simulink model "AA_Assemblage"  (R2020b)
settings: Solver=FixedStepAuto  StartTime=0.0  StopTime=inf  FixedStep=0.001  RelTol=1e-3
values from neighbouring files (symbols this model uses):
  smiData =     [A_robot_move.mat]
undefined symbols (not defined in the file or in its folder): Levenberg, Marquardt, W, X, Y, Z
libraries: sm_lib x1154, nesl_utility x40, robotlib x9, robotmaniplib x4, robotcorelib x2, simulink x1
(part 1 of 19)
settings Model: Creator=alessandrini  LastModifiedBy=alessandrini

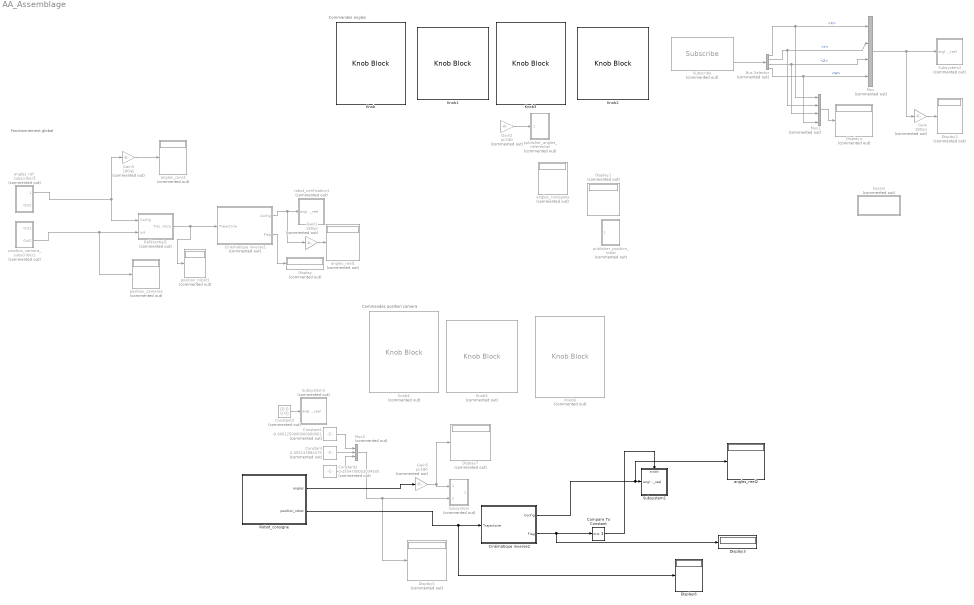
== system AA_Assemblage ==
  note: Fonctionnement global
  note: Commandes angles
  note: Commandes position camera
  Bus Selector : BusSelector  Commented=on  OutputSignals=X,Y,Z,W
  Cinématique inverse1 : Subsystem  Commented=on
  Cinématique inverse2 : Subsystem
  Compare To Constant : simulink/Logic and Bit Operations/Compare To Constant  relop===  const=1  OutDataTypeStr=boolean
  Constant : Constant  Commented=on  Value=0.055133984375
  Constant1 : Constant  Commented=on  Value=-0.0001250000000000001
  Constant2 : Constant  Commented=on  Value=0.1554700002034505
  Constant3 : Constant  Commented=on  Value=[0 0 0 0]
  Display{,1..2,4..5,7} (6 alike) : Display  Commented=on
  Display3 : Display
  Display6 : Display
  Gain : Gain  Commented=on  Gain=180/pi
  Gain1 : Gain  Commented=on  Gain=180/pi
  Gain2 : Gain  Commented=on  Gain=pi/180
  Gain3 : Gain  Commented=on  Gain=180/pi
  Gain5 : Gain  Commented=on  Gain=pi/180
  Knob : KnobBlock  ScaleMin=-30  ScaleMax=115
  Knob1 : KnobBlock  ScaleMin=-90  ScaleMax=45
  Knob2 : KnobBlock  ScaleMin=-60  ScaleMax=0
  Knob3 : KnobBlock  ScaleMin=-90  ScaleMax=20
  Knob4 : KnobBlock  Commented=on  ScaleMin=-0.01  ScaleMax=0.01
  Knob5 : KnobBlock  Commented=on  ScaleMin=0.05  ScaleMax=0.06
  Knob6 : KnobBlock  Commented=on  ScaleMin=0.15  ScaleMax=0.16
  Mux : Mux  Commented=on
  Mux1 : Mux  Commented=on
  Mux2 : Mux  Commented=on  Inputs=3
  Robot_consigne : Subsystem
  Référentiel1 : Subsystem  Commented=on
  Subscribe : robotlib/Subscribe  Commented=on  topicSource=Specify your own  topic=/angles_liaison  messageType=geometry_msgs/Quaternion  SampleTime=-1  legacyBusStruct=off  messageQueueLength=1
  Subsystem : Subsystem  Commented=on
  Subsystem1 : Subsystem
  Subsystem2 : Subsystem  Commented=on
  Subsystem3 : Subsystem  Commented=on
  angles_cons1 : Display  Commented=on
  angles_consignes : Display  Commented=on
  angles_reel1 : Display  Commented=on
  angles_reel2 : Display
  angles_ref_subscriber1 : Subsystem  Commented=on
  bassin : Subsystem  Commented=on  TreatAsAtomicUnit=on
  position_camera1 : Display  Commented=on
  position_camera_subscriber1 : Subsystem  Commented=on
  position_robot1 : Display  Commented=on
  publisher_angles_referentiel : Subsystem  Commented=on
  publisher_position_robot : Subsystem  Commented=on
  robot_verification1 : Subsystem  Commented=on
  wires:
  Gain1/1 -> angles_reel1/1
  Cinématique inverse1/2(Flag) -> Display/1
  Gain2/1 -> publisher_angles_referentiel/1(position)
  Cinématique inverse1/1(Config) -> Gain1/1, robot_verification1/1(angles_reel)
  Référentiel1/1(Trajectoire) -> Cinématique inverse1/1(Trajectoire), position_robot1/1
  position_camera_subscriber1/2(Out2) -> position_camera1/1, Référentiel1/2(In3)
  Gain3/1 -> angles_cons1/1
  angles_ref_subscriber1/1(Config) -> Gain3/1, Référentiel1/1(Config)
  Subscribe/2 -> Bus Selector/1
  Bus Selector/1 -> Mux1/1, Mux/1  "<X>"
  Bus Selector/4 -> Mux1/4, Mux/4  "<W>"
  Mux/1 -> Subsystem2/1(angles_reel), Gain/1
  Bus Selector/2 -> Mux/2, Mux1/2  "<Y>"
  Bus Selector/3 -> Mux/3, Mux1/3  "<Z>"
  Cinématique inverse2/1(Config) -> Subsystem1/1(angles_reel), angles_reel2/1
  Mux1/1 -> Display4/1
  Gain/1 -> Display2/1
  Cinématique inverse2/2(Flag) -> Display3/1, Compare To Constant/1
  Gain5/1 -> Display7/1, Subsystem/1(Config)
  Mux2/1 -> Display5/1, Subsystem/2(position)
  Constant/1 -> Mux2/2
  Constant1/1 -> Mux2/1
  Constant2/1 -> Mux2/3
  Constant3/1 -> Subsystem3/1(angles_reel)
  Robot_consigne/1(angles) -> Gain5/1
  Robot_consigne/2(position_robot) -> Display6/1, Cinématique inverse2/1(Trajectoire)
  Compare To Constant/1 -> Subsystem1/Enable

== system AA_Assemblage/Cinématique inverse1 ==
  Trajectoire : Inport
  Bus Selector : BusSelector  OutputSignals=ExitFlag
  Constant1 : Constant  Value=[0 0 0 1 1 1]  VectorParams1D=off
  Coordinate Transformation Conversion1 : robotcorelib/Coordinate Transformation Conversion  InputRepresentation=Translation Vector  InputEulerSequence=ZYX  ShowTrVecInputPort=on  OutputRepresentation=Homogeneous Transformation  OutputEulerSequence=ZYX  ShowTrVecOutputPort=on  SimulateUsing=Interpreted execution
  Delay : Delay  DelayLength=1  InitialCondition=([-45.92 243 205.5 63.6]*pi/180)'
  Inverse Kinematics : robotmaniplib/Inverse Kinematics  RigidBodyTree=robot  EndEffector=Body5  ShowInfo=on  SolverName=Levenberg-Marquardt  EnforceJointLimits=on  MaxIterations=1500  MaxTime=10  GradientTolerance=1e-7  SolutionTolerance=1e-6  StepTolerance=1e-14  ErrorChangeTolerance=1e-12  UseErrorDamping=on  DampingBias=0.0025  SimulateUsing=Interpreted execution
  Config : Outport
  Flag : Outport  Port=2
  wires:
  Coordinate Transformation Conversion1/1 -> Inverse Kinematics/1
  Delay/1 -> Inverse Kinematics/3
  Constant1/1 -> Inverse Kinematics/2
  Trajectoire/1 -> Coordinate Transformation Conversion1/1
  Inverse Kinematics/1 -> Delay/1, Config/1
  Inverse Kinematics/2 -> Bus Selector/1
  Bus Selector/1 -> Flag/1  "<ExitFlag>"

== system AA_Assemblage/Cinématique inverse2 ==
  Trajectoire : Inport
  Bus Selector : BusSelector  OutputSignals=ExitFlag
  Constant1 : Constant  Value=[0 0 0 1 1 1]  VectorParams1D=off
  Coordinate Transformation Conversion1 : robotcorelib/Coordinate Transformation Conversion  InputRepresentation=Translation Vector  InputEulerSequence=ZYX  ShowTrVecInputPort=on  OutputRepresentation=Homogeneous Transformation  OutputEulerSequence=ZYX  ShowTrVecOutputPort=on  SimulateUsing=Interpreted execution
  Delay1 : Delay  DelayLength=1  InitialCondition=([19 43 0 -30]*pi/180)'
  Inverse Kinematics : robotmaniplib/Inverse Kinematics  RigidBodyTree=robot  EndEffector=Body5  ShowInfo=on  SolverName=Levenberg-Marquardt  EnforceJointLimits=on  MaxIterations=1500  MaxTime=10  GradientTolerance=1e-7  SolutionTolerance=1e-6  StepTolerance=1e-14  ErrorChangeTolerance=1e-12  UseErrorDamping=on  DampingBias=0.0025  SimulateUsing=Interpreted execution
  Config : Outport
  Flag : Outport  Port=2
  wires:
  Coordinate Transformation Conversion1/1 -> Inverse Kinematics/1
  Delay1/1 -> Inverse Kinematics/3
  Constant1/1 -> Inverse Kinematics/2
  Trajectoire/1 -> Coordinate Transformation Conversion1/1
  Inverse Kinematics/1 -> Delay1/1, Config/1
  Inverse Kinematics/2 -> Bus Selector/1
  Bus Selector/1 -> Flag/1  "<ExitFlag>"

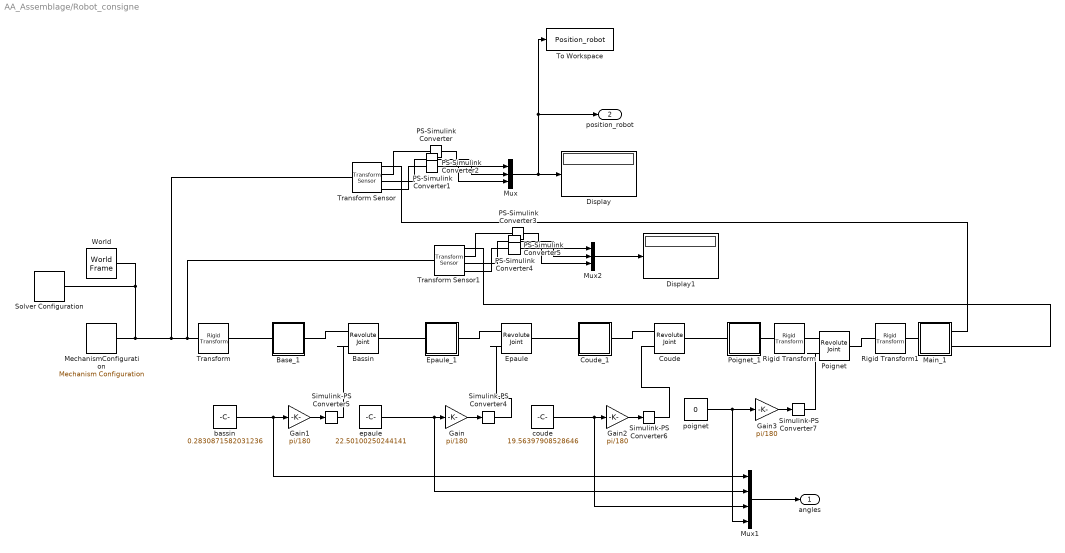
== system AA_Assemblage/Robot_consigne ==
  Base_1 : Subsystem
  Bassin : sm_lib/Joints/Revolute Joint  JointMode=Normal  SenseConstraintForce=off  SenseConstraintForceX=off  SenseConstraintForceY=off  SenseConstraintForceZ=off  SenseConstraintTorque=off  SenseConstraintTorqueX=off  SenseConstraintTorqueY=off  SenseConstraintTorqueZ=off  SenseTotalForce=off  SenseTotalForceX=off  SenseTotalForceY=off  SenseTotalForceZ=off  SenseTotalTorque=off  SenseTotalTorqueX=off  SenseTotalTorqueY=off  SenseTotalTorqueZ=off  CompositeWrenchDir=FollowerOnBase  CompositeWrenchFrame=BaseFrame  EquilibriumPosition=0  EquilibriumPositionUnits=deg  SpringStiffness=0  SpringStiffnessUnits=N*m/deg  DampingCoefficient=0  DampingCoefficientUnits=N*m/(deg/s)  TorqueActuationMode=ComputedTorque  MotionActuationMode=InputMotion  SensePosition=off  SenseVelocity=off  SenseAcceleration=off  SenseTorqueForce=off  SenseLowerLimitTorqueForce=off  SenseUpperLimitTorqueForce=off  LowerLimitSpecify=off  LowerLimitBound=-90  LowerLimitBoundUnits=deg  LowerLimitStiffness=1e4  LowerLimitStiffnessUnits=N*m/deg  LowerLimitDamping=10  LowerLimitDampingUnits=N*m/(deg/s)  LowerLimitTransitionRegionWidth=0.1  LowerLimitTransitionRegionWidthUnits=deg  UpperLimitSpecify=off  UpperLimitBound=90  UpperLimitBoundUnits=deg  UpperLimitStiffness=1e4  UpperLimitStiffnessUnits=N*m/deg  UpperLimitDamping=10  UpperLimitDampingUnits=N*m/(deg/s)  UpperLimitTransitionRegionWidth=0.1  UpperLimitTransitionRegionWidthUnits=deg  PositionTargetSpecify=on  PositionTargetPriority=Low  PositionTargetValue=smiData.RevoluteJoint(4).Rz.Pos  PositionTargetValueUnits=deg  VelocityTargetSpecify=off  VelocityTargetPriority=High  VelocityTargetValue=0  VelocityTargetValueUnits=deg/s
  Coude : sm_lib/Joints/Revolute Joint  JointMode=Normal  SenseConstraintForce=off  SenseConstraintForceX=off  SenseConstraintForceY=off  SenseConstraintForceZ=off  SenseConstraintTorque=off  SenseConstraintTorqueX=off  SenseConstraintTorqueY=off  SenseConstraintTorqueZ=off  SenseTotalForce=off  SenseTotalForceX=off  SenseTotalForceY=off  SenseTotalForceZ=off  SenseTotalTorque=off  SenseTotalTorqueX=off  SenseTotalTorqueY=off  SenseTotalTorqueZ=off  CompositeWrenchDir=FollowerOnBase  CompositeWrenchFrame=BaseFrame  EquilibriumPosition=0  EquilibriumPositionUnits=deg  SpringStiffness=0  SpringStiffnessUnits=N*m/deg  DampingCoefficient=0  DampingCoefficientUnits=N*m/(deg/s)  TorqueActuationMode=ComputedTorque  MotionActuationMode=InputMotion  SensePosition=off  SenseVelocity=off  SenseAcceleration=off  SenseTorqueForce=off  SenseLowerLimitTorqueForce=off  SenseUpperLimitTorqueForce=off  LowerLimitSpecify=off  LowerLimitBound=-90  LowerLimitBoundUnits=deg  LowerLimitStiffness=1e4  LowerLimitStiffnessUnits=N*m/deg  LowerLimitDamping=10  LowerLimitDampingUnits=N*m/(deg/s)  LowerLimitTransitionRegionWidth=0.1  LowerLimitTransitionRegionWidthUnits=deg  UpperLimitSpecify=off  UpperLimitBound=90  UpperLimitBoundUnits=deg  UpperLimitStiffness=1e4  UpperLimitStiffnessUnits=N*m/deg  UpperLimitDamping=10  UpperLimitDampingUnits=N*m/(deg/s)  UpperLimitTransitionRegionWidth=0.1  UpperLimitTransitionRegionWidthUnits=deg  PositionTargetSpecify=on  PositionTargetPriority=Low  PositionTargetValue=smiData.RevoluteJoint(1).Rz.Pos  PositionTargetValueUnits=deg  VelocityTargetSpecify=off  VelocityTargetPriority=High  VelocityTargetValue=0  VelocityTargetValueUnits=deg/s
  Coude_1 : Subsystem
  Display : Display
  Display1 : Display
  Epaule : sm_lib/Joints/Revolute Joint  JointMode=Normal  SenseConstraintForce=off  SenseConstraintForceX=off  SenseConstraintForceY=off  SenseConstraintForceZ=off  SenseConstraintTorque=off  SenseConstraintTorqueX=off  SenseConstraintTorqueY=off  SenseConstraintTorqueZ=off  SenseTotalForce=off  SenseTotalForceX=off  SenseTotalForceY=off  SenseTotalForceZ=off  SenseTotalTorque=off  SenseTotalTorqueX=off  SenseTotalTorqueY=off  SenseTotalTorqueZ=off  CompositeWrenchDir=FollowerOnBase  CompositeWrenchFrame=BaseFrame  EquilibriumPosition=0  EquilibriumPositionUnits=deg  SpringStiffness=0  SpringStiffnessUnits=N*m/deg  DampingCoefficient=0  DampingCoefficientUnits=N*m/(deg/s)  TorqueActuationMode=ComputedTorque  MotionActuationMode=InputMotion  SensePosition=off  SenseVelocity=off  SenseAcceleration=off  SenseTorqueForce=off  SenseLowerLimitTorqueForce=off  SenseUpperLimitTorqueForce=off  LowerLimitSpecify=off  LowerLimitBound=-90  LowerLimitBoundUnits=deg  LowerLimitStiffness=1e4  LowerLimitStiffnessUnits=N*m/deg  LowerLimitDamping=10  LowerLimitDampingUnits=N*m/(deg/s)  LowerLimitTransitionRegionWidth=0.1  LowerLimitTransitionRegionWidthUnits=deg  UpperLimitSpecify=off  UpperLimitBound=90  UpperLimitBoundUnits=deg  UpperLimitStiffness=1e4  UpperLimitStiffnessUnits=N*m/deg  UpperLimitDamping=10  UpperLimitDampingUnits=N*m/(deg/s)  UpperLimitTransitionRegionWidth=0.1  UpperLimitTransitionRegionWidthUnits=deg  PositionTargetSpecify=on  PositionTargetPriority=Low  PositionTargetValue=smiData.RevoluteJoint(3).Rz.Pos  PositionTargetValueUnits=deg  VelocityTargetSpecify=off  VelocityTargetPriority=High  VelocityTargetValue=0  VelocityTargetValueUnits=deg/s
  Epaule_1 : Subsystem
  Gain{,1..3} (4 alike) : Gain  Gain=pi/180
  Main_1 : Subsystem
  MechanismConfiguration : sm_lib/Utilities/Mechanism Configuration  UniformGravity=Constant  GravityVector=[0 0 -9.80665]  GravityVectorUnits=m/s^2  GravityUnits=m/s^2  LinearizationDelta=0.001  JointModeTransitionNonlinearIterations=2
  Mux : Mux  Inputs=3
  Mux1 : Mux
  Mux2 : Mux  Inputs=3
  PS-Simulink Converter{,1..5} (6 alike) : nesl_utility/PS-Simulink Converter  PhysicalDomain=network_engine_domain  SubClassName=ps_output  LeftPortType=input  RightPortType=output  PseudoPeriodic=off  Frequencies=[]  Unit=inherit  AffineConversion=off
  Poignet : sm_lib/Joints/Revolute Joint  JointMode=Normal  SenseConstraintForce=off  SenseConstraintForceX=off  SenseConstraintForceY=off  SenseConstraintForceZ=off  SenseConstraintTorque=off  SenseConstraintTorqueX=off  SenseConstraintTorqueY=off  SenseConstraintTorqueZ=off  SenseTotalForce=off  SenseTotalForceX=off  SenseTotalForceY=off  SenseTotalForceZ=off  SenseTotalTorque=off  SenseTotalTorqueX=off  SenseTotalTorqueY=off  SenseTotalTorqueZ=off  CompositeWrenchDir=FollowerOnBase  CompositeWrenchFrame=BaseFrame  EquilibriumPosition=0  EquilibriumPositionUnits=deg  SpringStiffness=0  SpringStiffnessUnits=N*m/deg  DampingCoefficient=0  DampingCoefficientUnits=N*m/(deg/s)  TorqueActuationMode=ComputedTorque  MotionActuationMode=InputMotion  SensePosition=off  SenseVelocity=off  SenseAcceleration=off  SenseTorqueForce=off  SenseLowerLimitTorqueForce=off  SenseUpperLimitTorqueForce=off  LowerLimitSpecify=off  LowerLimitBound=-90  LowerLimitBoundUnits=deg  LowerLimitStiffness=1e4  LowerLimitStiffnessUnits=N*m/deg  LowerLimitDamping=10  LowerLimitDampingUnits=N*m/(deg/s)  LowerLimitTransitionRegionWidth=0.1  LowerLimitTransitionRegionWidthUnits=deg  UpperLimitSpecify=off  UpperLimitBound=90  UpperLimitBoundUnits=deg  UpperLimitStiffness=1e4  UpperLimitStiffnessUnits=N*m/deg  UpperLimitDamping=10  UpperLimitDampingUnits=N*m/(deg/s)  UpperLimitTransitionRegionWidth=0.1  UpperLimitTransitionRegionWidthUnits=deg  PositionTargetSpecify=on  PositionTargetPriority=Low  PositionTargetValue=smiData.RevoluteJoint(2).Rz.Pos  PositionTargetValueUnits=deg  VelocityTargetSpecify=off  VelocityTargetPriority=High  VelocityTargetValue=0  VelocityTargetValueUnits=deg/s
  Poignet_1 : Subsystem
  Rigid Transform : sm_lib/Frames and Transforms/Rigid Transform  TranslationMethod=None  TranslationStandardOffset=0  TranslationLengthUnit=m  TranslationStandardAxis=+Z  TranslationCartesianOffset=[0 0 0]  TranslationROffset=0  TranslationROffsetUnits=m  TranslationZOffset=0  TranslationZOffsetUnits=m  TranslationThetaOffset=0  TranslationThetaOffsetUnits=deg  RotationMethod=ArbitraryAxis  RotationAngleUnits=deg  RotationStandardAxis=+Z  RotationAngle=180  RotationArbitraryAxis=[1 0 0]  FollAlignAxisA=+X  BaseAlignAxisA=+Y  FollAlignAxisB=+Y  BaseAlignAxisB=+Z  RotationSequenceAxes=FollowerAxes  RotationSequence=XYX  RotationSequenceAngles=[0 0 0]  RotationSequenceAnglesUnits=deg  RotationMatrix=[1 0 0; 0 1 0; 0 0 1]
  Rigid Transform1 : sm_lib/Frames and Transforms/Rigid Transform  TranslationMethod=None  TranslationStandardOffset=0  TranslationLengthUnit=m  TranslationStandardAxis=+Z  TranslationCartesianOffset=[0 0 0]  TranslationROffset=0  TranslationROffsetUnits=m  TranslationZOffset=0  TranslationZOffsetUnits=m  TranslationThetaOffset=0  TranslationThetaOffsetUnits=deg  RotationMethod=ArbitraryAxis  RotationAngleUnits=deg  RotationStandardAxis=+Z  RotationAngle=180  RotationArbitraryAxis=[1 0 0]  FollAlignAxisA=+X  BaseAlignAxisA=+Y  FollAlignAxisB=+Y  BaseAlignAxisB=+Z  RotationSequenceAxes=FollowerAxes  RotationSequence=XYX  RotationSequenceAngles=[0 0 0]  RotationSequenceAnglesUnits=deg  RotationMatrix=[1 0 0; 0 1 0; 0 0 1]
  Simulink-PS Converter{4..7} (4 alike) : nesl_utility/Simulink-PS Converter  PhysicalDomain=network_engine_domain  SubClassName=ps_input  LeftPortType=input  RightPortType=output  PseudoPeriodic=off  Frequencies=[]  NoiseDistribution=none  NoiseParameters=[]  Unit=1  AffineConversion=off  FilteringAndDerivatives=provide  SimscapeFilterOrder=1  InputFilterTimeConstant=0.001  UdotUserProvided=0
  Solver Configuration : nesl_utility/Solver Configuration  PhysicalDomain=network_engine_domain  SubClassName=solver  LeftPortType=input  RightPortType=generic  Tones=[]  Harmonics=[]  SimulateNoise=off  Profile=off  UseLocalSampling=off  EnableSwitchedLinearOptims=on  FrequencyDomain=off  UseCCode=off  RelTol=0.001  AbsTol=1e-06  MinStep=1e-09  ToWorkspace=off  RevertToSquareIcSolve=off  NumHomotopyIterations=100  PhasorMode=off  PhasorModeNumHarmonics=1  DoDC=off  ResidualTolerance=1e-09  UseLocalSolver=off  LocalSolverChoice=NE_BACKWARD_EULER_ADVANCER  LocalSolverSampleTime=0.001  DoFixedCost=off  MaxNonlinIter=3  MaxModeIter=2  ComputeImpulses=off  ImpulseIterations=2  LinearAlgebra=auto  EquationFormulation=NE_TIME_EF  DelaysMemoryBudget=1024  AutomaticFiltering=on  FilteringTimeConstant=0.001  PartitionStorageMethod=AS_NEEDED  PartitionMemoryBudget=1024  PartitionMethod=ROBUST
  To Workspace : ToWorkspace  VariableName=Position_robot  SaveFormat=Timeseries  SampleTime=-1
  Transform : sm_lib/Frames and Transforms/Rigid Transform  TranslationMethod=Cartesian  TranslationStandardOffset=0  TranslationLengthUnit=mm  TranslationStandardAxis=+Z  TranslationCartesianOffset=smiData.RigidTransform(104).translation  TranslationROffset=0  TranslationROffsetUnits=m  TranslationZOffset=0  TranslationZOffsetUnits=m  TranslationThetaOffset=0  TranslationThetaOffsetUnits=deg  RotationMethod=ArbitraryAxis  RotationAngleUnits=rad  RotationStandardAxis=+Z  RotationAngle=smiData.RigidTransform(104).angle  RotationArbitraryAxis=smiData.RigidTransform(104).axis  FollAlignAxisA=+X  BaseAlignAxisA=+Y  FollAlignAxisB=+Y  BaseAlignAxisB=+Z  RotationSequenceAxes=FollowerAxes  RotationSequence=XYX  RotationSequenceAngles=[0 0 0]  RotationSequenceAnglesUnits=deg  RotationMatrix=[1 0 0; 0 1 0; 0 0 1]
  Transform Sensor : sm_lib/Frames and Transforms/Transform Sensor  MeasurementFrame=World  SenseAngle=off  SenseAxis=off  SenseAngle1=off  SenseAngle2=off  SenseAngle3=off  SenseQ=off  SenseR=off  SenseOmegaX=off  SenseOmegaY=off  SenseOmegaZ=off  SenseOmega1=off  SenseOmega2=off  SenseOmega3=off  SenseQDot=off  SenseRDot=off  SenseAlphaX=off  SenseAlphaY=off  SenseAlphaZ=off  SenseAlpha1=off  SenseAlpha2=off  SenseAlpha3=off  SenseQDDot=off  SenseRDDot=off  SenseX=on  SenseY=on  SenseZ=on  SenseRad=off  SenseAzim=off  SenseDist=off  SenseInc=off  SenseXDot=off  SenseYDot=off  SenseZDot=off  SenseRadDot=off  SenseAzimDot=off  SenseDistDot=off  SenseIncDot=off  SenseXDDot=off  SenseYDDot=off  SenseZDDot=off  SenseRadDDot=off  SenseAzimDDot=off  SenseDistDDot=off  SenseIncDDot=off
  Transform Sensor1 : sm_lib/Frames and Transforms/Transform Sensor  MeasurementFrame=World  SenseAngle=off  SenseAxis=off  SenseAngle1=off  SenseAngle2=off  SenseAngle3=off  SenseQ=off  SenseR=off  SenseOmegaX=off  SenseOmegaY=off  SenseOmegaZ=off  SenseOmega1=off  SenseOmega2=off  SenseOmega3=off  SenseQDot=off  SenseRDot=off  SenseAlphaX=off  SenseAlphaY=off  SenseAlphaZ=off  SenseAlpha1=off  SenseAlpha2=off  SenseAlpha3=off  SenseQDDot=off  SenseRDDot=off  SenseX=on  SenseY=on  SenseZ=on  SenseRad=off  SenseAzim=off  SenseDist=off  SenseInc=off  SenseXDot=off  SenseYDot=off  SenseZDot=off  SenseRadDot=off  SenseAzimDot=off  SenseDistDot=off  SenseIncDot=off  SenseXDDot=off  SenseYDDot=off  SenseZDDot=off  SenseRadDDot=off  SenseAzimDDot=off  SenseDistDDot=off  SenseIncDDot=off
  World : sm_lib/Frames and Transforms/World Frame
  bassin : Constant  Value=0.2830871582031236
  coude : Constant  Value=19.56397908528646
  epaule : Constant  Value=22.50100250244141
  poignet : Constant  Value=0
  angles : Outport
  position_robot : Outport  Port=2
  wires:
  poignet/1 -> Gain3/1, Mux1/4
  bassin/1 -> Mux1/1, Gain1/1
  coude/1 -> Mux1/3, Gain2/1
  Gain/1 -> Simulink-PS Converter4/1
  Gain3/1 -> Simulink-PS Converter7/1
  Gain2/1 -> Simulink-PS Converter6/1
  Gain1/1 -> Simulink-PS Converter5/1
  Mux1/1 -> angles/1
  epaule/1 -> Mux1/2, Gain/1
  PS-Simulink Converter1/1 -> Mux/2
  PS-Simulink Converter/1 -> Mux/1
  PS-Simulink Converter2/1 -> Mux/3
  Mux/1 -> To Workspace/1, position_robot/1, Display/1
  PS-Simulink Converter3/1 -> Mux2/1
  PS-Simulink Converter5/1 -> Mux2/3
  PS-Simulink Converter4/1 -> Mux2/2
  Mux2/1 -> Display1/1
  connections:
  Transform Sensor/LConn1 -- MechanismConfiguration/RConn1 -- Solver Configuration/RConn1 -- World/RConn1 -- Transform Sensor1/LConn1 -- Transform/LConn1
  Transform/RConn1 -- Base_1/LConn1
  Coude/LConn2 -- Simulink-PS Converter6/RConn1
  Base_1/RConn1 -- Bassin/LConn1
  PS-Simulink Converter2/LConn1 -- Transform Sensor/RConn4
  Bassin/LConn2 -- Simulink-PS Converter5/RConn1
  Transform Sensor/RConn1 -- Main_1/RConn1
  PS-Simulink Converter/LConn1 -- Transform Sensor/RConn2
  Poignet/LConn2 -- Simulink-PS Converter7/RConn1
  Poignet/LConn1 -- Rigid Transform/RConn1
  Rigid Transform1/LConn1 -- Poignet/RConn1
  Coude_1/LConn1 -- Epaule/RConn1
  Epaule/LConn1 -- Epaule_1/RConn1
  PS-Simulink Converter1/LConn1 -- Transform Sensor/RConn3
  Coude/LConn1 -- Coude_1/RConn1
  Epaule/LConn2 -- Simulink-PS Converter4/RConn1
  Bassin/RConn1 -- Epaule_1/LConn1
  Coude/RConn1 -- Poignet_1/LConn1
  Main_1/LConn1 -- Rigid Transform1/RConn1
  Rigid Transform/LConn1 -- Poignet_1/RConn1
  PS-Simulink Converter4/LConn1 -- Transform Sensor1/RConn3
  PS-Simulink Converter5/LConn1 -- Transform Sensor1/RConn4
  Main_1/RConn2 -- Transform Sensor1/RConn1
  PS-Simulink Converter3/LConn1 -- Transform Sensor1/RConn2

== system AA_Assemblage/Référentiel1 ==
  Config : Inport
  In3 : Inport  Port=2
  Constant4 : Constant
  Get Transform : robotmaniplib/Get Transform  RigidBodyTree=robot  SourceBody=Body5  TargetBody=Base  SimulateUsing=Interpreted execution
  Mux2 : Mux  Inputs=2
  Product : Product  Multiplication=Matrix(*)
  Selector : Selector  InputPortWidth=4  IndexOptions=Starting index (dialog)  Indices=1  OutputSizes=3
  Trajectoire : Outport
  wires:
  Config/1 -> Get Transform/1
  Constant4/1 -> Mux2/2
  Product/1 -> Selector/1
  In3/1 -> Mux2/1
  Selector/1 -> Trajectoire/1
  Get Transform/1 -> Product/1
  Mux2/1 -> Product/2

== system AA_Assemblage/Subsystem ==
  Config : Inport
  position : Inport  Port=2
  Constant : Constant
  Get Transform : robotmaniplib/Get Transform  RigidBodyTree=robot  SourceBody=Body6  TargetBody=Base  SimulateUsing=Interpreted execution
  Mux : Mux  Inputs=2
  Product : Product  Multiplication=Matrix(*)
  Selector : Selector  InputPortWidth=4  IndexOptions=Starting index (dialog)  Indices=[1]  OutputSizes=3
  Trajectoire : Outport
  wires:
  Selector/1 -> Trajectoire/1
  Product/1 -> Selector/1
  Config/1 -> Get Transform/1
  Get Transform/1 -> Product/1
  position/1 -> Mux/1
  Constant/1 -> Mux/2
  Mux/1 -> Product/2

== system AA_Assemblage/Subsystem1 ==
  note: robot_verification
  angles_reel : Inport
  Enable : EnablePort
  Demux : Demux
  Robot_verif : Subsystem
  Simulink-PS Converter{,1..3} (4 alike) : nesl_utility/Simulink-PS Converter  PhysicalDomain=network_engine_domain  SubClassName=ps_input  LeftPortType=input  RightPortType=output  PseudoPeriodic=off  Frequencies=[]  NoiseDistribution=none  NoiseParameters=[]  Unit=1  AffineConversion=off  FilteringAndDerivatives=filter  SimscapeFilterOrder=2  InputFilterTimeConstant=0.001  UdotUserProvided=0
  wires:
  Demux/2 -> Simulink-PS Converter1/1  "epaule"
  angles_reel/1 -> Demux/1
  Demux/4 -> Simulink-PS Converter3/1  "poignet"
  Demux/1 -> Simulink-PS Converter/1  "bassin"
  Demux/3 -> Simulink-PS Converter2/1  "coude"
  connections:
  Simulink-PS Converter2/RConn1 -- Robot_verif/LConn3
  Simulink-PS Converter1/RConn1 -- Robot_verif/LConn2
  Simulink-PS Converter3/RConn1 -- Robot_verif/LConn4
  Simulink-PS Converter/RConn1 -- Robot_verif/LConn1

== system AA_Assemblage/Subsystem2 ==
  note: robot_verification
  angles_reel : Inport
  Demux : Demux
  Robot_verif : Subsystem
  Simulink-PS Converter{,1..3} (4 alike) : nesl_utility/Simulink-PS Converter  PhysicalDomain=network_engine_domain  SubClassName=ps_input  LeftPortType=input  RightPortType=output  PseudoPeriodic=off  Frequencies=[]  NoiseDistribution=none  NoiseParameters=[]  Unit=1  AffineConversion=off  FilteringAndDerivatives=filter  SimscapeFilterOrder=2  InputFilterTimeConstant=0.001  UdotUserProvided=0
  wires:
  Demux/2 -> Simulink-PS Converter1/1  "epaule"
  angles_reel/1 -> Demux/1
  Demux/4 -> Simulink-PS Converter3/1  "poignet"
  Demux/1 -> Simulink-PS Converter/1  "bassin"
  Demux/3 -> Simulink-PS Converter2/1  "coude"
  connections:
  Simulink-PS Converter2/RConn1 -- Robot_verif/LConn3
  Simulink-PS Converter1/RConn1 -- Robot_verif/LConn2
  Simulink-PS Converter3/RConn1 -- Robot_verif/LConn4
  Simulink-PS Converter/RConn1 -- Robot_verif/LConn1

== system AA_Assemblage/Subsystem3 ==
  note: robot_verification
  angles_reel : Inport
  Demux : Demux
  Robot_verif : Subsystem
  Simulink-PS Converter{,1..3} (4 alike) : nesl_utility/Simulink-PS Converter  PhysicalDomain=network_engine_domain  SubClassName=ps_input  LeftPortType=input  RightPortType=output  PseudoPeriodic=off  Frequencies=[]  NoiseDistribution=none  NoiseParameters=[]  Unit=1  AffineConversion=off  FilteringAndDerivatives=filter  SimscapeFilterOrder=2  InputFilterTimeConstant=0.001  UdotUserProvided=0
  wires:
  Demux/2 -> Simulink-PS Converter1/1  "epaule"
  angles_reel/1 -> Demux/1
  Demux/4 -> Simulink-PS Converter3/1  "poignet"
  Demux/1 -> Simulink-PS Converter/1  "bassin"
  Demux/3 -> Simulink-PS Converter2/1  "coude"
  connections:
  Simulink-PS Converter2/RConn1 -- Robot_verif/LConn3
  Simulink-PS Converter1/RConn1 -- Robot_verif/LConn2
  Simulink-PS Converter3/RConn1 -- Robot_verif/LConn4
  Simulink-PS Converter/RConn1 -- Robot_verif/LConn1

== system AA_Assemblage/angles_ref_subscriber1 ==
  Bus Selector : BusSelector  OutputSignals=X,Y,Z,W
  Mux1 : Mux
  Subscribe : robotlib/Subscribe  topicSource=Specify your own  topic=/angles_ref  messageType=geometry_msgs/Quaternion  SampleTime=-1  legacyBusStruct=off  messageQueueLength=1
  Config : Outport
  Out2 : Outport  Port=2
  wires:
  Subscribe/2 -> Bus Selector/1
  Bus Selector/1 -> Mux1/1  "<X>"
  Bus Selector/2 -> Mux1/2  "<Y>"
  Mux1/1 -> Config/1
  Bus Selector/3 -> Mux1/3  "<Z>"
  Subscribe/1 -> Out2/1
  Bus Selector/4 -> Mux1/4  "<W>"

== system AA_Assemblage/bassin ==
  Add : Sum
  Constant : Constant  Value=-30
  For Iterator : ForIterator  ResetStates=reset  IterationLimit=7
  Gain : Gain  Gain=20
  epaule : Subsystem  TreatAsAtomicUnit=on
  wires:
  Constant/1 -> Add/2
  Add/1 -> epaule/1(In1)
  Gain/1 -> Add/1
  For Iterator/1 -> Gain/1

== system AA_Assemblage/position_camera_subscriber1 ==
  Bus Selector1 : BusSelector  OutputSignals=X,Y,Z
  Mux2 : Mux  Inputs=3
  Subscribe1 : robotlib/Subscribe  topicSource=Specify your own  topic=/position_camera  messageType=geometry_msgs/Point  SampleTime=-1  legacyBusStruct=off  messageQueueLength=1
  Out1 : Outport
  Out2 : Outport  Port=2
  wires:
  Bus Selector1/2 -> Mux2/2  "<Y>"
  Bus Selector1/1 -> Mux2/1  "<X>"
  Subscribe1/2 -> Bus Selector1/1
  Subscribe1/1 -> Out1/1
  Mux2/1 -> Out2/1
  Bus Selector1/3 -> Mux2/3  "<Z>"

== system AA_Assemblage/publisher_angles_referentiel ==
  position : Inport
  Blank Message1 : robotlib/Blank Message  messageClass=Message  entityType=geometry_msgs/Quaternion  messageType=geometry_msgs/Quaternion  SampleTime=inf  legacyBusStruct=off
  Bus Assignment : BusAssignment  AssignedSignals=X,Y,Z,W
  Demux : Demux
  Publish : robotlib/Publish  topicSource=Specify your own  topic=/angles_referentiel  messageType=geometry_msgs/Quaternion  legacyBusStruct=off  messageQueueLength=1
  wires:
  Demux/2 -> Bus Assignment/3
  Bus Assignment/1 -> Publish/1
  Demux/1 -> Bus Assignment/2
  Blank Message1/1 -> Bus Assignment/1
  position/1 -> Demux/1
  Demux/3 -> Bus Assignment/4
  Demux/4 -> Bus Assignment/5

== system AA_Assemblage/publisher_position_robot ==
  position : Inport
  Blank Message1 : robotlib/Blank Message  messageClass=Message  entityType=geometry_msgs/Point  messageType=geometry_msgs/Point  SampleTime=inf  legacyBusStruct=off
  Bus Assignment : BusAssignment  AssignedSignals=X,Y,Z
  Demux : Demux  Outputs=3
  Publish : robotlib/Publish  topicSource=Specify your own  topic=/position_robot  messageType=geometry_msgs/Point  legacyBusStruct=off  messageQueueLength=1
  wires:
  Demux/2 -> Bus Assignment/3
  Bus Assignment/1 -> Publish/1
  Demux/1 -> Bus Assignment/2
  Blank Message1/1 -> Bus Assignment/1
  position/1 -> Demux/1
  Demux/3 -> Bus Assignment/4

== system AA_Assemblage/robot_verification1 ==
  note: robot verification
  angles_reel : Inport
  Demux : Demux
  Robot_verif : Subsystem
  Simulink-PS Converter{,1..3} (4 alike) : nesl_utility/Simulink-PS Converter  PhysicalDomain=network_engine_domain  SubClassName=ps_input  LeftPortType=input  RightPortType=output  PseudoPeriodic=off  Frequencies=[]  NoiseDistribution=none  NoiseParameters=[]  Unit=1  AffineConversion=off  FilteringAndDerivatives=filter  SimscapeFilterOrder=2  InputFilterTimeConstant=0.001  UdotUserProvided=0
  wires:
  Demux/3 -> Simulink-PS Converter2/1  "coude"
  Demux/1 -> Simulink-PS Converter/1  "bassin"
  Demux/4 -> Simulink-PS Converter3/1  "poignet"
  angles_reel/1 -> Demux/1
  Demux/2 -> Simulink-PS Converter1/1  "epaule"
  connections:
  Simulink-PS Converter/RConn1 -- Robot_verif/LConn1
  Simulink-PS Converter3/RConn1 -- Robot_verif/LConn4
  Simulink-PS Converter1/RConn1 -- Robot_verif/LConn2
  Simulink-PS Converter2/RConn1 -- Robot_verif/LConn3

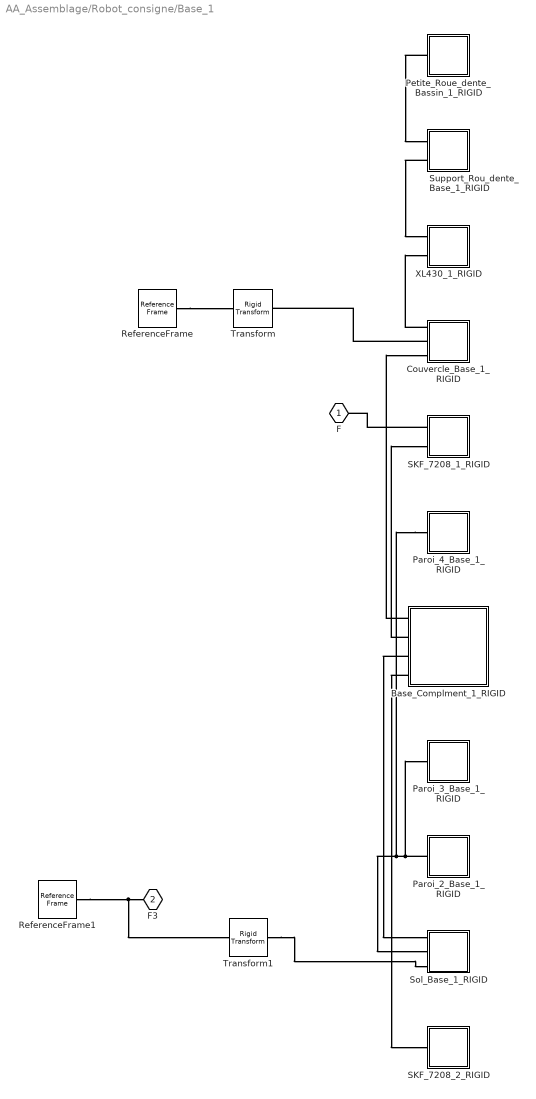
== system AA_Assemblage/Robot_consigne/Base_1 ==
  Base_Complment_1_RIGID : Subsystem
  Couvercle_Base_1_RIGID : Subsystem
  Paroi_2_Base_1_RIGID : Subsystem
  Paroi_3_Base_1_RIGID : Subsystem
  Paroi_4_Base_1_RIGID : Subsystem
  Petite_Roue_dente_Bassin_1_RIGID : Subsystem
  ReferenceFrame : sm_lib/Frames and Transforms/Reference Frame
  ReferenceFrame1 : sm_lib/Frames and Transforms/Reference Frame
  SKF_7208_1_RIGID : Subsystem
  SKF_7208_2_RIGID : Subsystem
  Sol_Base_1_RIGID : Subsystem
  Support_Rou_dente_Base_1_RIGID : Subsystem
  Transform : sm_lib/Frames and Transforms/Rigid Transform  TranslationMethod=Cartesian  TranslationStandardOffset=0  TranslationLengthUnit=mm  TranslationStandardAxis=+Z  TranslationCartesianOffset=smiData.RigidTransform(103).translation  TranslationROffset=0  TranslationROffsetUnits=m  TranslationZOffset=0  TranslationZOffsetUnits=m  TranslationThetaOffset=0  TranslationThetaOffsetUnits=deg  RotationMethod=ArbitraryAxis  RotationAngleUnits=rad  RotationStandardAxis=+Z  RotationAngle=smiData.RigidTransform(103).angle  RotationArbitraryAxis=smiData.RigidTransform(103).axis  FollAlignAxisA=+X  BaseAlignAxisA=+Y  FollAlignAxisB=+Y  BaseAlignAxisB=+Z  RotationSequenceAxes=FollowerAxes  RotationSequence=XYX  RotationSequenceAngles=[0 0 0]  RotationSequenceAnglesUnits=deg  RotationMatrix=[1 0 0; 0 1 0; 0 0 1]
  Transform1 : sm_lib/Frames and Transforms/Rigid Transform  TranslationMethod=Cartesian  TranslationStandardOffset=0  TranslationLengthUnit=mm  TranslationStandardAxis=+Z  TranslationCartesianOffset=smiData.RigidTransform(106).translation  TranslationROffset=0  TranslationROffsetUnits=m  TranslationZOffset=0  TranslationZOffsetUnits=m  TranslationThetaOffset=0  TranslationThetaOffsetUnits=deg  RotationMethod=ArbitraryAxis  RotationAngleUnits=rad  RotationStandardAxis=+Z  RotationAngle=smiData.RigidTransform(106).angle  RotationArbitraryAxis=smiData.RigidTransform(106).axis  FollAlignAxisA=+X  BaseAlignAxisA=+Y  FollAlignAxisB=+Y  BaseAlignAxisB=+Z  RotationSequenceAxes=FollowerAxes  RotationSequence=XYX  RotationSequenceAngles=[0 0 0]  RotationSequenceAnglesUnits=deg  RotationMatrix=[1 0 0; 0 1 0; 0 0 1]
  XL430_1_RIGID : Subsystem
  F : PMIOPort  Side=Right
  F3 : PMIOPort  Port=2  Side=Left
  connections:
  Paroi_4_Base_1_RIGID/LConn1 -- Sol_Base_1_RIGID/LConn2 -- Paroi_2_Base_1_RIGID/LConn1 -- Paroi_3_Base_1_RIGID/LConn1
  Support_Rou_dente_Base_1_RIGID/LConn2 -- XL430_1_RIGID/LConn1
  ReferenceFrame/RConn1 -- Transform/LConn1
  Couvercle_Base_1_RIGID/LConn1 -- XL430_1_RIGID/LConn2
  Base_Complment_1_RIGID/LConn3 -- Sol_Base_1_RIGID/LConn1
  Petite_Roue_dente_Bassin_1_RIGID/LConn1 -- Support_Rou_dente_Base_1_RIGID/LConn1
  Base_Complment_1_RIGID/LConn1 -- Couvercle_Base_1_RIGID/LConn3
  Base_Complment_1_RIGID/LConn2 -- SKF_7208_1_RIGID/LConn2
  Base_Complment_1_RIGID/LConn4 -- SKF_7208_2_RIGID/LConn1
  SKF_7208_1_RIGID/LConn1 -- F/RConn1
  Couvercle_Base_1_RIGID/LConn2 -- Transform/RConn1
  F3/RConn1 -- Transform1/LConn1 -- ReferenceFrame1/RConn1
  Transform1/RConn1 -- Sol_Base_1_RIGID/LConn3

== system AA_Assemblage/Robot_consigne/Coude_1 ==
  Adaptateur_Arbre_01_1_RIGID : Subsystem
  Arbre_1_1_RIGID : Subsystem
  Bras_1_droite_1_RIGID : Subsystem
  Bras_1_gauche_1_RIGID : Subsystem
  Grande_Roue_dente_paule_1_RIGID : Subsystem
  Petite_Roue_dente_Coude_1_RIGID : Subsystem
  ReferenceFrame : sm_lib/Frames and Transforms/Reference Frame
  SKF_7202_1_RIGID : Subsystem
  SKF_7202_2_RIGID : Subsystem
  Support_Rou_dente_coude_et_poignet_1_RIGID : Subsystem
  XL430_1_RIGID : Subsystem
  F1 : PMIOPort  Side=Left
  F : PMIOPort  Port=2  Side=Right
  connections:
  Bras_1_droite_1_RIGID/LConn2 -- SKF_7202_1_RIGID/LConn2
  Bras_1_droite_1_RIGID/LConn1 -- XL430_1_RIGID/LConn2
  Adaptateur_Arbre_01_1_RIGID/LConn2 -- F1/RConn1
  Arbre_1_1_RIGID/LConn2 -- Bras_1_droite_1_RIGID/LConn3
  Support_Rou_dente_coude_et_poignet_1_RIGID/LConn2 -- XL430_1_RIGID/LConn1
  Adaptateur_Arbre_01_1_RIGID/LConn3 -- Grande_Roue_dente_paule_1_RIGID/LConn1
  Arbre_1_1_RIGID/LConn1 -- Bras_1_gauche_1_RIGID/LConn2
  Adaptateur_Arbre_01_1_RIGID/LConn1 -- Arbre_1_1_RIGID/LConn3
  Bras_1_gauche_1_RIGID/LConn1 -- SKF_7202_2_RIGID/LConn1
  Petite_Roue_dente_Coude_1_RIGID/LConn1 -- Support_Rou_dente_coude_et_poignet_1_RIGID/LConn1
  SKF_7202_1_RIGID/LConn1 -- F/RConn1

== system AA_Assemblage/Robot_consigne/Epaule_1 ==
  Bras_01_droite_3_RIGID : Subsystem
  Bras_01_gauche_4_RIGID : Subsystem
  Mt_1_RIGID : Subsystem
  Part_2_1_RIGID : Subsystem
  Petite_Roue_dente_paule_1_RIGID : Subsystem
  Plateau_complmentaire_du_mt_2_RIGID : Subsystem
  ReferenceFrame : sm_lib/Frames and Transforms/Reference Frame
  SKF_7202_1_RIGID : Subsystem
  SKF_7202_2_RIGID : Subsystem
  XL430_1_RIGID : Subsystem
  F1 : PMIOPort  Side=Left
  F : PMIOPort  Port=2  Side=Right
  connections:
  Petite_Roue_dente_paule_1_RIGID/LConn1 -- XL430_1_RIGID/LConn1
  Mt_1_RIGID/LConn5 -- Part_2_1_RIGID/LConn1
  Bras_01_gauche_4_RIGID/LConn3 -- Mt_1_RIGID/LConn2
  Mt_1_RIGID/LConn4 -- Plateau_complmentaire_du_mt_2_RIGID/LConn1
  Bras_01_droite_3_RIGID/LConn2 -- Mt_1_RIGID/LConn1
  Bras_01_gauche_4_RIGID/LConn1 -- XL430_1_RIGID/LConn2
  Bras_01_gauche_4_RIGID/LConn2 -- SKF_7202_2_RIGID/LConn1
  Bras_01_droite_3_RIGID/LConn1 -- SKF_7202_1_RIGID/LConn2
  SKF_7202_1_RIGID/LConn1 -- F/RConn1
  Mt_1_RIGID/LConn3 -- F1/RConn1

== system AA_Assemblage/Robot_consigne/Main_1 ==
  Arbre_Poignet_1_RIGID : Subsystem
  Main_assemble_1 : Subsystem
  Poignet_1_RIGID : Subsystem
  engrenage_sortie_1_RIGID : Subsystem
  F : PMIOPort  Side=Left
  F1 : PMIOPort  Port=2  Side=Right
  F2 : PMIOPort  Port=3  Side=Right
  connections:
  Arbre_Poignet_1_RIGID/LConn3 -- engrenage_sortie_1_RIGID/LConn1
  Main_assemble_1/LConn1 -- Poignet_1_RIGID/LConn1
  Arbre_Poignet_1_RIGID/LConn1 -- Poignet_1_RIGID/LConn2
  Arbre_Poignet_1_RIGID/LConn2 -- F/RConn1
  F1/RConn1 -- Main_assemble_1/RConn1
  F2/RConn1 -- Main_assemble_1/RConn2

== system AA_Assemblage/Robot_consigne/Poignet_1 ==
  Bras1_1_RIGID : Subsystem
  Grande_Roue_dente_Coude_1_RIGID : Subsystem
  Part_1_1_RIGID : Subsystem
  Part_2_1_RIGID : Subsystem
  ReferenceFrame : sm_lib/Frames and Transforms/Reference Frame
  SKF_7202_1_RIGID : Subsystem
  SKF_7202_2_RIGID : Subsystem
  Support_Rou_dente_coude_et_poignet_1_RIGID : Subsystem
  XL430_1_RIGID : Subsystem
  F : PMIOPort  Side=Left
  F1 : PMIOPort  Port=2  Side=Right
  connections:
  Bras1_1_RIGID/LConn3 -- SKF_7202_1_RIGID/LConn1
  Bras1_1_RIGID/LConn2 -- Part_1_1_RIGID/LConn3
  Part_1_1_RIGID/LConn4 -- Part_2_1_RIGID/LConn1
  Grande_Roue_dente_Coude_1_RIGID/LConn1 -- Part_1_1_RIGID/LConn1
  Bras1_1_RIGID/LConn1 -- XL430_1_RIGID/LConn2
  Part_2_1_RIGID/LConn2 -- SKF_7202_2_RIGID/LConn1
  Support_Rou_dente_coude_et_poignet_1_RIGID/LConn1 -- XL430_1_RIGID/LConn1
  Part_1_1_RIGID/LConn2 -- F/RConn1
  SKF_7202_2_RIGID/LConn2 -- F1/RConn1

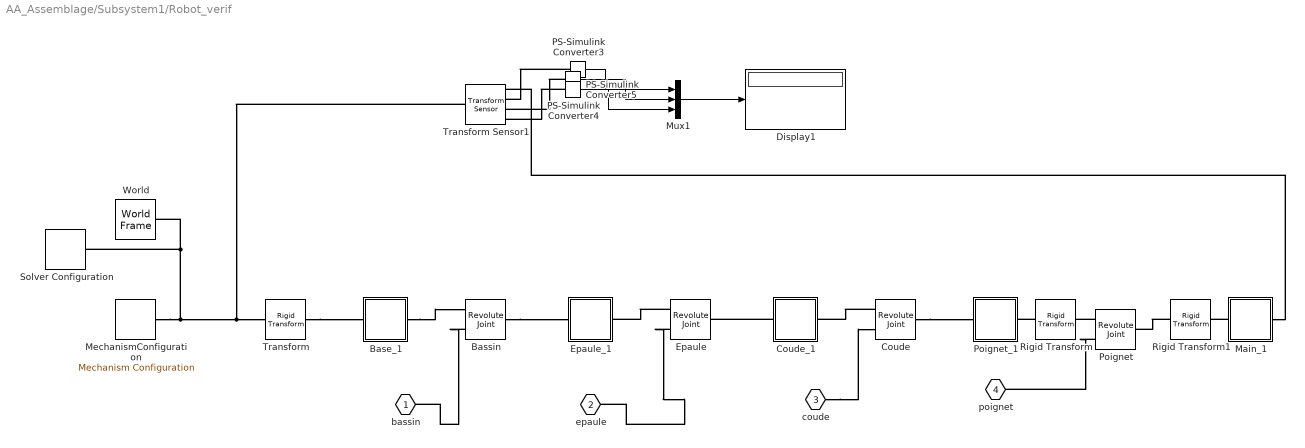
== system AA_Assemblage/Subsystem1/Robot_verif ==
  Base_1 : Subsystem
  Bassin : sm_lib/Joints/Revolute Joint  JointMode=Normal  SenseConstraintForce=off  SenseConstraintForceX=off  SenseConstraintForceY=off  SenseConstraintForceZ=off  SenseConstraintTorque=off  SenseConstraintTorqueX=off  SenseConstraintTorqueY=off  SenseConstraintTorqueZ=off  SenseTotalForce=off  SenseTotalForceX=off  SenseTotalForceY=off  SenseTotalForceZ=off  SenseTotalTorque=off  SenseTotalTorqueX=off  SenseTotalTorqueY=off  SenseTotalTorqueZ=off  CompositeWrenchDir=FollowerOnBase  CompositeWrenchFrame=BaseFrame  EquilibriumPosition=0  EquilibriumPositionUnits=deg  SpringStiffness=0  SpringStiffnessUnits=N*m/deg  DampingCoefficient=0  DampingCoefficientUnits=N*m/(deg/s)  TorqueActuationMode=ComputedTorque  MotionActuationMode=InputMotion  SensePosition=off  SenseVelocity=off  SenseAcceleration=off  SenseTorqueForce=off  SenseLowerLimitTorqueForce=off  SenseUpperLimitTorqueForce=off  LowerLimitSpecify=off  LowerLimitBound=-90  LowerLimitBoundUnits=deg  LowerLimitStiffness=1e4  LowerLimitStiffnessUnits=N*m/deg  LowerLimitDamping=10  LowerLimitDampingUnits=N*m/(deg/s)  LowerLimitTransitionRegionWidth=0.1  LowerLimitTransitionRegionWidthUnits=deg  UpperLimitSpecify=off  UpperLimitBound=90  UpperLimitBoundUnits=deg  UpperLimitStiffness=1e4  UpperLimitStiffnessUnits=N*m/deg  UpperLimitDamping=10  UpperLimitDampingUnits=N*m/(deg/s)  UpperLimitTransitionRegionWidth=0.1  UpperLimitTransitionRegionWidthUnits=deg  PositionTargetSpecify=on  PositionTargetPriority=Low  PositionTargetValue=smiData.RevoluteJoint(4).Rz.Pos  PositionTargetValueUnits=deg  VelocityTargetSpecify=off  VelocityTargetPriority=High  VelocityTargetValue=0  VelocityTargetValueUnits=deg/s
  Coude : sm_lib/Joints/Revolute Joint  JointMode=Normal  SenseConstraintForce=off  SenseConstraintForceX=off  SenseConstraintForceY=off  SenseConstraintForceZ=off  SenseConstraintTorque=off  SenseConstraintTorqueX=off  SenseConstraintTorqueY=off  SenseConstraintTorqueZ=off  SenseTotalForce=off  SenseTotalForceX=off  SenseTotalForceY=off  SenseTotalForceZ=off  SenseTotalTorque=off  SenseTotalTorqueX=off  SenseTotalTorqueY=off  SenseTotalTorqueZ=off  CompositeWrenchDir=FollowerOnBase  CompositeWrenchFrame=BaseFrame  EquilibriumPosition=0  EquilibriumPositionUnits=deg  SpringStiffness=0  SpringStiffnessUnits=N*m/deg  DampingCoefficient=0  DampingCoefficientUnits=N*m/(deg/s)  TorqueActuationMode=ComputedTorque  MotionActuationMode=InputMotion  SensePosition=off  SenseVelocity=off  SenseAcceleration=off  SenseTorqueForce=off  SenseLowerLimitTorqueForce=off  SenseUpperLimitTorqueForce=off  LowerLimitSpecify=off  LowerLimitBound=-90  LowerLimitBoundUnits=deg  LowerLimitStiffness=1e4  LowerLimitStiffnessUnits=N*m/deg  LowerLimitDamping=10  LowerLimitDampingUnits=N*m/(deg/s)  LowerLimitTransitionRegionWidth=0.1  LowerLimitTransitionRegionWidthUnits=deg  UpperLimitSpecify=off  UpperLimitBound=90  UpperLimitBoundUnits=deg  UpperLimitStiffness=1e4  UpperLimitStiffnessUnits=N*m/deg  UpperLimitDamping=10  UpperLimitDampingUnits=N*m/(deg/s)  UpperLimitTransitionRegionWidth=0.1  UpperLimitTransitionRegionWidthUnits=deg  PositionTargetSpecify=on  PositionTargetPriority=Low  PositionTargetValue=smiData.RevoluteJoint(1).Rz.Pos  PositionTargetValueUnits=deg  VelocityTargetSpecify=off  VelocityTargetPriority=High  VelocityTargetValue=0  VelocityTargetValueUnits=deg/s
  Coude_1 : Subsystem
  Display1 : Display
  Epaule : sm_lib/Joints/Revolute Joint  JointMode=Normal  SenseConstraintForce=off  SenseConstraintForceX=off  SenseConstraintForceY=off  SenseConstraintForceZ=off  SenseConstraintTorque=off  SenseConstraintTorqueX=off  SenseConstraintTorqueY=off  SenseConstraintTorqueZ=off  SenseTotalForce=off  SenseTotalForceX=off  SenseTotalForceY=off  SenseTotalForceZ=off  SenseTotalTorque=off  SenseTotalTorqueX=off  SenseTotalTorqueY=off  SenseTotalTorqueZ=off  CompositeWrenchDir=FollowerOnBase  CompositeWrenchFrame=BaseFrame  EquilibriumPosition=0  EquilibriumPositionUnits=deg  SpringStiffness=0  SpringStiffnessUnits=N*m/deg  DampingCoefficient=0  DampingCoefficientUnits=N*m/(deg/s)  TorqueActuationMode=ComputedTorque  MotionActuationMode=InputMotion  SensePosition=off  SenseVelocity=off  SenseAcceleration=off  SenseTorqueForce=off  SenseLowerLimitTorqueForce=off  SenseUpperLimitTorqueForce=off  LowerLimitSpecify=off  LowerLimitBound=-90  LowerLimitBoundUnits=deg  LowerLimitStiffness=1e4  LowerLimitStiffnessUnits=N*m/deg  LowerLimitDamping=10  LowerLimitDampingUnits=N*m/(deg/s)  LowerLimitTransitionRegionWidth=0.1  LowerLimitTransitionRegionWidthUnits=deg  UpperLimitSpecify=off  UpperLimitBound=90  UpperLimitBoundUnits=deg  UpperLimitStiffness=1e4  UpperLimitStiffnessUnits=N*m/deg  UpperLimitDamping=10  UpperLimitDampingUnits=N*m/(deg/s)  UpperLimitTransitionRegionWidth=0.1  UpperLimitTransitionRegionWidthUnits=deg  PositionTargetSpecify=on  PositionTargetPriority=Low  PositionTargetValue=smiData.RevoluteJoint(3).Rz.Pos  PositionTargetValueUnits=deg  VelocityTargetSpecify=off  VelocityTargetPriority=High  VelocityTargetValue=0  VelocityTargetValueUnits=deg/s
  Epaule_1 : Subsystem
  Main_1 : Subsystem
  MechanismConfiguration : sm_lib/Utilities/Mechanism Configuration  UniformGravity=Constant  GravityVector=[0 0 -9.80665]  GravityVectorUnits=m/s^2  GravityUnits=m/s^2  LinearizationDelta=0.001  JointModeTransitionNonlinearIterations=2
  Mux1 : Mux  Inputs=3
  PS-Simulink Converter3 : nesl_utility/PS-Simulink Converter  PhysicalDomain=network_engine_domain  SubClassName=ps_output  LeftPortType=input  RightPortType=output  PseudoPeriodic=off  Frequencies=[]  Unit=inherit  AffineConversion=off
  PS-Simulink Converter4 : nesl_utility/PS-Simulink Converter  PhysicalDomain=network_engine_domain  SubClassName=ps_output  LeftPortType=input  RightPortType=output  PseudoPeriodic=off  Frequencies=[]  Unit=inherit  AffineConversion=off
  PS-Simulink Converter5 : nesl_utility/PS-Simulink Converter  PhysicalDomain=network_engine_domain  SubClassName=ps_output  LeftPortType=input  RightPortType=output  PseudoPeriodic=off  Frequencies=[]  Unit=inherit  AffineConversion=off
  Poignet : sm_lib/Joints/Revolute Joint  JointMode=Normal  SenseConstraintForce=off  SenseConstraintForceX=off  SenseConstraintForceY=off  SenseConstraintForceZ=off  SenseConstraintTorque=off  SenseConstraintTorqueX=off  SenseConstraintTorqueY=off  SenseConstraintTorqueZ=off  SenseTotalForce=off  SenseTotalForceX=off  SenseTotalForceY=off  SenseTotalForceZ=off  SenseTotalTorque=off  SenseTotalTorqueX=off  SenseTotalTorqueY=off  SenseTotalTorqueZ=off  CompositeWrenchDir=FollowerOnBase  CompositeWrenchFrame=BaseFrame  EquilibriumPosition=0  EquilibriumPositionUnits=deg  SpringStiffness=0  SpringStiffnessUnits=N*m/deg  DampingCoefficient=0  DampingCoefficientUnits=N*m/(deg/s)  TorqueActuationMode=ComputedTorque  MotionActuationMode=InputMotion  SensePosition=off  SenseVelocity=off  SenseAcceleration=off  SenseTorqueForce=off  SenseLowerLimitTorqueForce=off  SenseUpperLimitTorqueForce=off  LowerLimitSpecify=off  LowerLimitBound=-90  LowerLimitBoundUnits=deg  LowerLimitStiffness=1e4  LowerLimitStiffnessUnits=N*m/deg  LowerLimitDamping=10  LowerLimitDampingUnits=N*m/(deg/s)  LowerLimitTransitionRegionWidth=0.1  LowerLimitTransitionRegionWidthUnits=deg  UpperLimitSpecify=off  UpperLimitBound=90  UpperLimitBoundUnits=deg  UpperLimitStiffness=1e4  UpperLimitStiffnessUnits=N*m/deg  UpperLimitDamping=10  UpperLimitDampingUnits=N*m/(deg/s)  UpperLimitTransitionRegionWidth=0.1  UpperLimitTransitionRegionWidthUnits=deg  PositionTargetSpecify=on  PositionTargetPriority=Low  PositionTargetValue=smiData.RevoluteJoint(2).Rz.Pos  PositionTargetValueUnits=deg  VelocityTargetSpecify=off  VelocityTargetPriority=High  VelocityTargetValue=0  VelocityTargetValueUnits=deg/s
  Poignet_1 : Subsystem
  Rigid Transform : sm_lib/Frames and Transforms/Rigid Transform  TranslationMethod=None  TranslationStandardOffset=0  TranslationLengthUnit=m  TranslationStandardAxis=+Z  TranslationCartesianOffset=[0 0 0]  TranslationROffset=0  TranslationROffsetUnits=m  TranslationZOffset=0  TranslationZOffsetUnits=m  TranslationThetaOffset=0  TranslationThetaOffsetUnits=deg  RotationMethod=ArbitraryAxis  RotationAngleUnits=deg  RotationStandardAxis=+Z  RotationAngle=180  RotationArbitraryAxis=[1 0 0]  FollAlignAxisA=+X  BaseAlignAxisA=+Y  FollAlignAxisB=+Y  BaseAlignAxisB=+Z  RotationSequenceAxes=FollowerAxes  RotationSequence=XYX  RotationSequenceAngles=[0 0 0]  RotationSequenceAnglesUnits=deg  RotationMatrix=[1 0 0; 0 1 0; 0 0 1]
  Rigid Transform1 : sm_lib/Frames and Transforms/Rigid Transform  TranslationMethod=None  TranslationStandardOffset=0  TranslationLengthUnit=m  TranslationStandardAxis=+Z  TranslationCartesianOffset=[0 0 0]  TranslationROffset=0  TranslationROffsetUnits=m  TranslationZOffset=0  TranslationZOffsetUnits=m  TranslationThetaOffset=0  TranslationThetaOffsetUnits=deg  RotationMethod=ArbitraryAxis  RotationAngleUnits=deg  RotationStandardAxis=+Z  RotationAngle=180  RotationArbitraryAxis=[1 0 0]  FollAlignAxisA=+X  BaseAlignAxisA=+Y  FollAlignAxisB=+Y  BaseAlignAxisB=+Z  RotationSequenceAxes=FollowerAxes  RotationSequence=XYX  RotationSequenceAngles=[0 0 0]  RotationSequenceAnglesUnits=deg  RotationMatrix=[1 0 0; 0 1 0; 0 0 1]
  Solver Configuration : nesl_utility/Solver Configuration  PhysicalDomain=network_engine_domain  SubClassName=solver  LeftPortType=input  RightPortType=generic  Tones=[]  Harmonics=[]  SimulateNoise=off  Profile=off  UseLocalSampling=off  EnableSwitchedLinearOptims=on  FrequencyDomain=off  UseCCode=off  RelTol=0.001  AbsTol=1e-06  MinStep=1e-09  ToWorkspace=off  RevertToSquareIcSolve=off  NumHomotopyIterations=100  PhasorMode=off  PhasorModeNumHarmonics=1  DoDC=off  ResidualTolerance=1e-09  UseLocalSolver=off  LocalSolverChoice=NE_BACKWARD_EULER_ADVANCER  LocalSolverSampleTime=0.001  DoFixedCost=off  MaxNonlinIter=3  MaxModeIter=2  ComputeImpulses=off  ImpulseIterations=2  LinearAlgebra=auto  EquationFormulation=NE_TIME_EF  DelaysMemoryBudget=1024  AutomaticFiltering=on  FilteringTimeConstant=0.001  PartitionStorageMethod=AS_NEEDED  PartitionMemoryBudget=1024  PartitionMethod=ROBUST
  Transform : sm_lib/Frames and Transforms/Rigid Transform  TranslationMethod=Cartesian  TranslationStandardOffset=0  TranslationLengthUnit=mm  TranslationStandardAxis=+Z  TranslationCartesianOffset=smiData.RigidTransform(104).translation  TranslationROffset=0  TranslationROffsetUnits=m  TranslationZOffset=0  TranslationZOffsetUnits=m  TranslationThetaOffset=0  TranslationThetaOffsetUnits=deg  RotationMethod=ArbitraryAxis  RotationAngleUnits=rad  RotationStandardAxis=+Z  RotationAngle=smiData.RigidTransform(104).angle  RotationArbitraryAxis=smiData.RigidTransform(104).axis  FollAlignAxisA=+X  BaseAlignAxisA=+Y  FollAlignAxisB=+Y  BaseAlignAxisB=+Z  RotationSequenceAxes=FollowerAxes  RotationSequence=XYX  RotationSequenceAngles=[0 0 0]  RotationSequenceAnglesUnits=deg  RotationMatrix=[1 0 0; 0 1 0; 0 0 1]
  Transform Sensor1 : sm_lib/Frames and Transforms/Transform Sensor  MeasurementFrame=World  SenseAngle=off  SenseAxis=off  SenseAngle1=off  SenseAngle2=off  SenseAngle3=off  SenseQ=off  SenseR=off  SenseOmegaX=off  SenseOmegaY=off  SenseOmegaZ=off  SenseOmega1=off  SenseOmega2=off  SenseOmega3=off  SenseQDot=off  SenseRDot=off  SenseAlphaX=off  SenseAlphaY=off  SenseAlphaZ=off  SenseAlpha1=off  SenseAlpha2=off  SenseAlpha3=off  SenseQDDot=off  SenseRDDot=off  SenseX=on  SenseY=on  SenseZ=on  SenseRad=off  SenseAzim=off  SenseDist=off  SenseInc=off  SenseXDot=off  SenseYDot=off  SenseZDot=off  SenseRadDot=off  SenseAzimDot=off  SenseDistDot=off  SenseIncDot=off  SenseXDDot=off  SenseYDDot=off  SenseZDDot=off  SenseRadDDot=off  SenseAzimDDot=off  SenseDistDDot=off  SenseIncDDot=off
  World : sm_lib/Frames and Transforms/World Frame
  bassin : PMIOPort  Side=Left
  epaule : PMIOPort  Port=2  Side=Left
  coude : PMIOPort  Port=3  Side=Left
  poignet : PMIOPort  Port=4  Side=Left
  wires:
  PS-Simulink Converter5/1 -> Mux1/3
  PS-Simulink Converter3/1 -> Mux1/1
  Mux1/1 -> Display1/1
  PS-Simulink Converter4/1 -> Mux1/2
  connections:
  World/RConn1 -- Solver Configuration/RConn1 -- MechanismConfiguration/RConn1 -- Transform Sensor1/LConn1 -- Transform/LConn1
  Bassin/RConn1 -- Epaule_1/LConn1
  Coude_1/LConn1 -- Epaule/RConn1
  Epaule/LConn2 -- epaule/RConn1
  Coude/RConn1 -- Poignet_1/LConn1
  Main_1/LConn1 -- Rigid Transform1/RConn1
  Coude/LConn1 -- Coude_1/RConn1
  Rigid Transform/LConn1 -- Poignet_1/RConn1
  Epaule/LConn1 -- Epaule_1/RConn1
  Rigid Transform1/LConn1 -- Poignet/RConn1
  Poignet/LConn2 -- poignet/RConn1
  Base_1/RConn1 -- Bassin/LConn1
  coude/RConn1 -- Coude/LConn2
  Bassin/LConn2 -- bassin/RConn1
  Poignet/LConn1 -- Rigid Transform/RConn1
  Transform/RConn1 -- Base_1/LConn1
  PS-Simulink Converter5/LConn1 -- Transform Sensor1/RConn4
  PS-Simulink Converter3/LConn1 -- Transform Sensor1/RConn2
  PS-Simulink Converter4/LConn1 -- Transform Sensor1/RConn3
  Main_1/RConn1 -- Transform Sensor1/RConn1
